simulink model "LQR_WIP"  (R2024b)
settings: Solver=FixedStepAuto  StartTime=0.0  StopTime=0.3  FixedStep=0.005  RelTol=1e-3  EnableMultiTasking=on
values from neighbouring files (symbols this model uses):
  K = lqr(A, B, Q, R)    [IP_Simulations.m]
undefined symbols (not defined in the file or in its folder): Discrete, Time
libraries: arduinolib x4, ctrlSharedLib x2, arduinosensorlib x1
settings Model: ExtModeTrigDuration=2  Creator=jitendra  LastModifiedBy=alexcullen
settings SolverCC: AlgebraicLoopSolver=TrustRegion  AutoInsertRateTranBlk=on
settings DataIOCC: ExternalInput=getinputstruct(op_trim1)  InitialState=getstatestruct(op_trim1)  ReturnWorkspaceOutputs=off
settings OptimizationCC: EnhancedBackFolding=on  PassReuseOutputArgsAs=Individual arguments  ZeroExternalMemoryAtStartup=off  ZeroInternalMemoryAtStartup=off  MaxStackSize=64  OptimizeBlockOrder=speed  DifferentSizesBufferReuse=on  OptimizationCustomize=off  EfficientTunableParamExpr=on
settings DebuggingCC: ParameterTunabilityLossMsg=error  UnconnectedInputMsg=warning  UnconnectedOutputMsg=warning  UnconnectedLineMsg=warning  ArithmeticOperatorsInVariantConditions=warning
settings HardwareCC: ProdBitPerInt=16  ProdBitPerPointer=16  ProdBitPerSizeT=16  ProdBitPerPtrDiffT=16  ProdLargestAtomicFloat=None  ProdWordSize=8  ProdHWDeviceType=Atmel->AVR
settings ModelReferenceCC: EnableRefExpFcnMdlSchedulingChecks=on
settings SFSimCC: SimUseLocalCustomCode=off  MATLABDynamicMemAlloc=off  CustomCodeUndefinedFunction=UseInterfaceOnly
settings RTWCC: Description=Embedded Coder  SystemTargetFile=ert.tlc  HardwareBoard=Arduino Uno  TemplateMakefile=ert_default_tmf  RTWUseLocalCustomCode=off  Toolchain=Arduino AVR  BuildConfiguration=Faster Runs  GPUComputeCapability=3.5
settings CodeAppCC: ForceParamTrailComments=on  IgnoreCustomStorageClasses=off  OperatorAnnotations=on  SimulinkDataObjDesc=on  SFDataObjDesc=on  InsertBlockDesc=on
settings ERTTargetCC: SupportContinuousTime=on  SupportVariableSizeSignals=on  ExtModeTransport=3  ExtModeStaticAlloc=on  ExtModeAutomaticAllocSize=off  ExtModeStaticAllocSize=250  ExtModeMexFile=ext_xcp  ExtModeIntrfLevel=Level2 - Open  InlinedParameterPlacement=Hierarchical

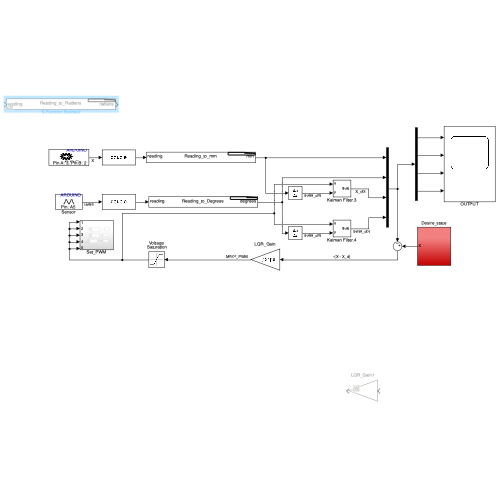
[thumbnail: Simulink's stored preview of the top-level diagram]
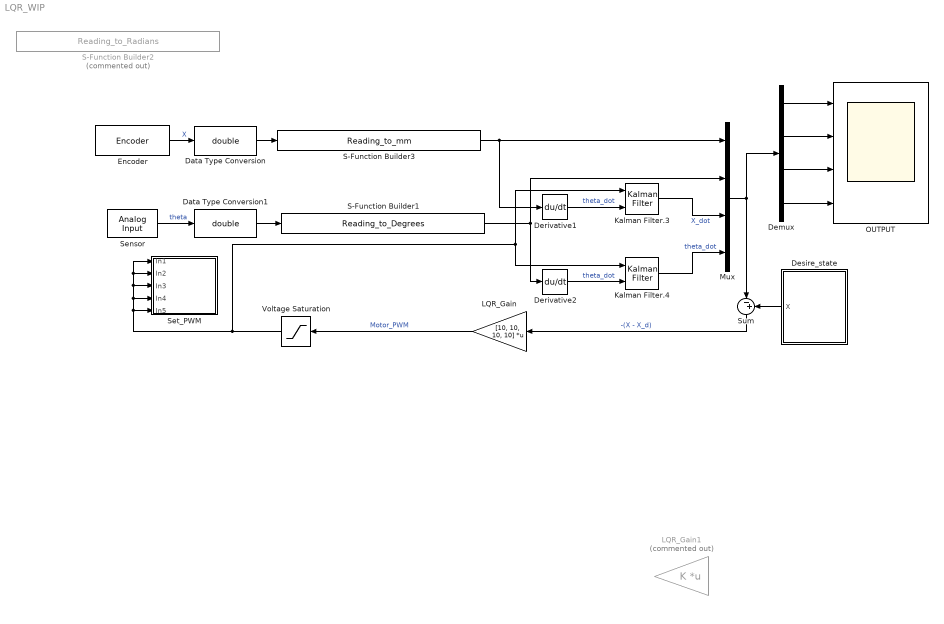
== system LQR_WIP ==
  Data Type Conversion : DataTypeConversion  OutDataTypeStr=double  SaturateOnIntegerOverflow=off  RndMeth=Floor
  Data Type Conversion1 : DataTypeConversion  OutDataTypeStr=double  SaturateOnIntegerOverflow=off  RndMeth=Floor
  Demux : Demux
  Derivative1 : Derivative
  Derivative2 : Derivative
  Desire_state : Subsystem
  Encoder : arduinosensorlib/Encoder  InputA=3  InputB=2  Mode=No reset  SampleTime=0.005
  Kalman Filter.3 : ctrlSharedLib/Kalman Filter  TimeDomain=Discrete-Time  UseCurrentEstimator=on  ModelSource=LTI State-Space Variable  ModelSourceVariable=ss(0.95,1,1,0,1)  A=0.95  B=1  C=1  D=0  NumberOfStates=1  NumberOfInputs=1  NumberOfOutputs=1  InitialEstimateSource=Dialog  X0=0  P0=10  UseK=off  UseGH=off  NumberOfProcessNoiseInputs=1  G=1  TimeInvariantG=on  H=0  TimeInvariantH=on  Q=0.05  TimeInvariantQ=on  R=1  TimeInvariantR=on  N=0  TimeInvariantN=on  AddInputPort=on  AddEnablePort=off  OutputEstimatedY=off  OutputP=off  Ts=-1
  Kalman Filter.4 : ctrlSharedLib/Kalman Filter  TimeDomain=Discrete-Time  UseCurrentEstimator=on  ModelSource=LTI State-Space Variable  ModelSourceVariable=ss(0.95,1,1,0,1)  A=0.95  B=1  C=1  D=0  NumberOfStates=1  NumberOfInputs=1  NumberOfOutputs=1  InitialEstimateSource=Dialog  X0=0  P0=10  UseK=off  UseGH=off  NumberOfProcessNoiseInputs=1  G=1  TimeInvariantG=on  H=0  TimeInvariantH=on  Q=0.05  TimeInvariantQ=on  R=1  TimeInvariantR=on  N=0  TimeInvariantN=on  AddInputPort=on  AddEnablePort=off  OutputEstimatedY=off  OutputP=off  Ts=-1
  LQR_Gain : Gain  Gain=[10, 10, 10, 10]  Multiplication=Matrix(K*u)
  LQR_Gain1 : Gain  Commented=on  Gain=K  Multiplication=Matrix(K*u)
  Mux : Mux
  OUTPUT : Scope  NumInputPorts=4
  S-Function Builder1 : S-Function  FunctionName=Reading_to_Degrees  SFunctionModules=Reading_to_Degrees_wrapper.c  SFunctionDeploymentMode=off  EnableBusSupport=off  mask(S-Function Builder){}
      mask help: Simulink:masks:SFunctionBuilder_MD
      mask init:
      | val = [[.9  0.75 0.75 1 1 .9 .9 1]',[1 1 0.75 0.75 .9 .9 1 .9]'];try , sys = get_param(gcb,'SfunBuilderFcnName');if isempty(sys), sys = get_param(gcb,'FunctionName'); end,catch, sys = get_param(gcb,'FunctionName'); end
      settings: CopyFcn=set_param(gcbh,'LinkStatus','none')  OpenFcn=sfunctionwizard(gcbh)
      mask Display: plot(val(:,1),val(:,2)),disp(sys),port_label('input',1,'reading'),port_label('output',1,'degrees')
  S-Function Builder2 : S-Function  Commented=on  FunctionName=Reading_to_Radians  SFunctionModules=Reading_to_Radians_wrapper.c  SFunctionDeploymentMode=off  EnableBusSupport=off  mask(S-Function Builder){}
      mask help: Simulink:masks:SFunctionBuilder_MD
      mask init: same as LQR_WIP/S-Function Builder1
      settings: CopyFcn=set_param(gcbh,'LinkStatus','none')  OpenFcn=sfunctionwizard(gcbh)
      mask Display:
      | plot(val(:,1),val(:,2))
      | disp(sys)
      | port_label('input',1,sprintf('%s', 'reading'),'interpreter','tex')
      | port_label('output',1,sprintf('%s', 'radians'),'interpreter','tex')
  S-Function Builder3 : S-Function  FunctionName=Reading_to_mm  SFunctionModules=Reading_to_mm_wrapper.c  SFunctionDeploymentMode=off  EnableBusSupport=off  mask(S-Function Builder){}
      mask help: Simulink:masks:SFunctionBuilder_MD
      mask init: same as LQR_WIP/S-Function Builder1
      settings: CopyFcn=set_param(gcbh,'LinkStatus','none')  OpenFcn=sfunctionwizard(gcbh)
      mask Display: plot(val(:,1),val(:,2)),disp(sys),port_label('input',1,'reading'),port_label('output',1,'mm')
  Sensor : arduinolib/Analog Input  pinNumber=5  ReadResultsOnly=off  ConversionTriggerSource=Software  ExternalTriggerType=uint32( 0 )  OutputDataType=uint16  EnableConversionCompleteNotify=off  EnableOuputStatus=off  SampleTime=0.005  blockPlatform=arduino
  Set_PWM : Subsystem
  Sum : Sum  Inputs=|-+
  Voltage Saturation : Saturate  UpperLimit=255  LowerLimit=-255
  wires:
  Kalman Filter.3/1 -> Mux/3  "X_dot"
  Kalman Filter.4/1 -> Mux/4  "theta_dot"
  Mux/1 -> Sum/1, Demux/1
  LQR_Gain/1 -> Voltage Saturation/1  "Motor_PWM"
  Desire_state/1(X) -> Sum/2
  Sum/1 -> LQR_Gain/1  "-(X - X_d)"
  Demux/1 -> OUTPUT/1
  Demux/3 -> OUTPUT/3
  Demux/2 -> OUTPUT/2
  Demux/4 -> OUTPUT/4
  Voltage Saturation/1 -> Kalman Filter.3/1, Kalman Filter.4/1, Set_PWM/1(In1), Set_PWM/2(In2), Set_PWM/3(In3), Set_PWM/4(In4), Set_PWM/5(In5)
  Sensor/1 -> Data Type Conversion1/1  "theta"
  Data Type Conversion1/1 -> S-Function Builder1/1
  S-Function Builder1/1 -> Derivative2/1, Mux/2
  Encoder/1 -> Data Type Conversion/1  "X"
  Derivative2/1 -> Kalman Filter.4/2  "theta_dot"
  Derivative1/1 -> Kalman Filter.3/2  "theta_dot"
  Data Type Conversion/1 -> S-Function Builder3/1
  S-Function Builder3/1 -> Mux/1, Derivative1/1

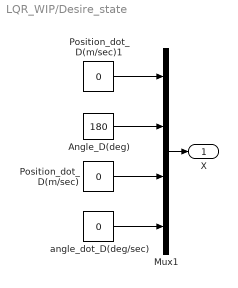
== system LQR_WIP/Desire_state ==
  Angle_D(deg) : Constant  Value=180
  Mux1 : Mux
  Position_dot_D(m/sec) : Constant  Value=0
  Position_dot_D(m/sec)1 : Constant  Value=0
  angle_dot_D(deg/sec) : Constant  Value=0
  X : Outport  VectorParamsAs1DForOutWhenUnconnected=off
  wires:
  Mux1/1 -> X/1
  Position_dot_D(m/sec)/1 -> Mux1/3
  angle_dot_D(deg/sec)/1 -> Mux1/4
  Angle_D(deg)/1 -> Mux1/2
  Position_dot_D(m/sec)1/1 -> Mux1/1

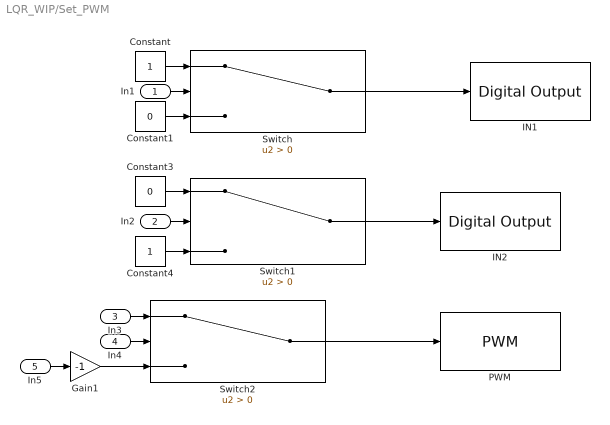
== system LQR_WIP/Set_PWM ==
  In1 : Inport
  In2 : Inport  Port=2
  In3 : Inport  Port=3
  In4 : Inport  Port=4
  In5 : Inport  Port=5
  Constant : Constant
  Constant1 : Constant  Value=0
  Constant3 : Constant  Value=0
  Constant4 : Constant
  Gain1 : Gain  Gain=-1
  IN1 : arduinolib/Digital Output  pinNumber=10  Direction=output  blockPlatform=arduino
  IN2 : arduinolib/Digital Output  pinNumber=11  Direction=output  blockPlatform=arduino
  PWM : arduinolib/PWM  pinNumber=9  frequencyType=Default  desiredFrequency=255  achievableFrequency=254.9963
  Switch : Switch  Criteria=u2 > Threshold  SaturateOnIntegerOverflow=off  InputSameDT=off
  Switch1 : Switch  Criteria=u2 > Threshold  SaturateOnIntegerOverflow=off  InputSameDT=off
  Switch2 : Switch  Criteria=u2 > Threshold  SaturateOnIntegerOverflow=off  InputSameDT=off
  wires:
  In1/1 -> Switch/2
  Switch2/1 -> PWM/1
  Switch/1 -> IN1/1
  Switch1/1 -> IN2/1
  Constant1/1 -> Switch/3
  In2/1 -> Switch1/2
  Constant3/1 -> Switch1/1
  In5/1 -> Gain1/1
  In4/1 -> Switch2/2
  Gain1/1 -> Switch2/3
  Constant/1 -> Switch/1
  In3/1 -> Switch2/1
  Constant4/1 -> Switch1/3
